simulink model "Ex10"  (R2019b)
settings: Solver=VariableStepAuto  StartTime=0.0  StopTime=20  RelTol=1e-3
values from neighbouring files (symbols this model uses):
  A = 1    [Ex_10.m]    (also in Ex_20.m = 0.1; Ex_28.m = Vf*Wn^2; Ex_29.m = 0.01)
  D = D_v(i)    [Ex_10.m]    (also in Ex_20.m = 3000; Ex_22.m = 0.4; Ex_23.m = 0.1; Ex_29.m = 0.1)
  K = 1    [Ex_10.m]    (also in Ex_21.m; Ex_22.m; Ex_24.m = 1 / qsi^2; Ex_31.m = 4.26)
  M = 1    [Ex_10.m]    (also in Ex_22.m = 5)
settings Model: Creator=andre  LastModifiedBy=andre

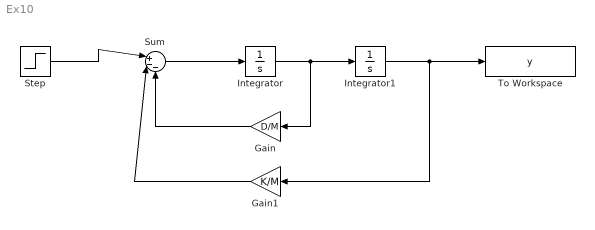
== system Ex10 ==
  Gain : Gain  Gain=D/M
  Gain1 : Gain  Gain=K/M
  Integrator : Integrator
  Integrator1 : Integrator
  Step : Step  Time=0  After=A  SampleTime=0
  Sum : Sum  Inputs=|+--
  To Workspace : ToWorkspace  VariableName=y  SaveFormat=Timeseries  SampleTime=-1
  wires:
  Integrator/1 -> Gain/1, Integrator1/1
  Sum/1 -> Integrator/1
  Integrator1/1 -> To Workspace/1, Gain1/1
  Gain/1 -> Sum/3
  Gain1/1 -> Sum/2
  Step/1 -> Sum/1
